simulink subsystem "ClusteringAlgoTemplate"  (R2022b)
settings: Solver=VariableStepAuto  StartTime=0.0  StopTime=10.0  RelTol=1e-3
settings Model: Creator=smryk  LastModifiedBy=smryk

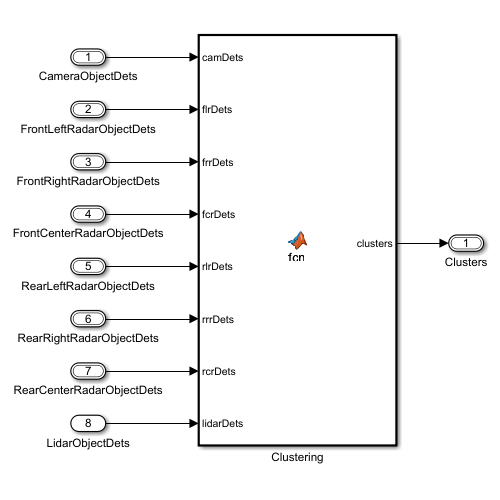
[thumbnail: Simulink's stored preview of the top-level diagram]
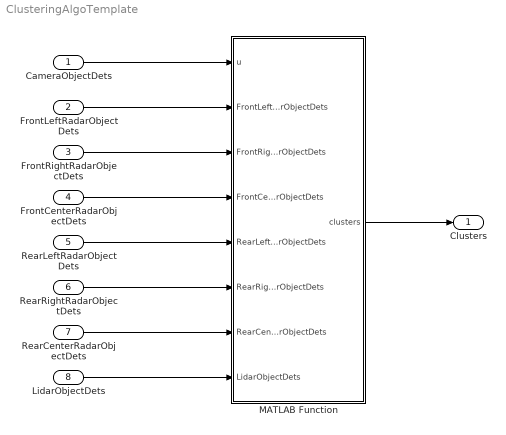
== system ClusteringAlgoTemplate ==
  CameraObjectDets : Inport  OutDataTypeStr=Bus: BusObjectDetections1
  FrontLeftRadarObjectDets : Inport  Port=2  OutDataTypeStr=Bus: BusDrivingRadarDataGenerator1
  FrontRightRadarObjectDets : Inport  Port=3  OutDataTypeStr=Bus: BusDrivingRadarDataGenerator1
  FrontCenterRadarObjectDets : Inport  Port=4  OutDataTypeStr=Bus: BusDrivingRadarDataGenerator1
  RearLeftRadarObjectDets : Inport  Port=5  OutDataTypeStr=Bus: BusDrivingRadarDataGenerator1
  RearRightRadarObjectDets : Inport  Port=6  OutDataTypeStr=Bus: BusDrivingRadarDataGenerator1
  RearCenterRadarObjectDets : Inport  Port=7  OutDataTypeStr=Bus: BusDrivingRadarDataGenerator1
  LidarObjectDets : Inport  Port=8
  MATLAB Function : MATLAB Function  TreatAsAtomicUnit=on
  Clusters : Outport  OutDataTypeStr=Bus: BusObjectDetections1
  wires:
  LidarObjectDets/1 -> MATLAB Function/8(LidarObjectDets)
  RearCenterRadarObjectDets/1 -> MATLAB Function/7(RearCenterRadarObjectDets)
  RearRightRadarObjectDets/1 -> MATLAB Function/6(RearRightRadarObjectDets)
  RearLeftRadarObjectDets/1 -> MATLAB Function/5(RearLeftRadarObjectDets)
  FrontCenterRadarObjectDets/1 -> MATLAB Function/4(FrontCenterRadarObjectDets)
  FrontRightRadarObjectDets/1 -> MATLAB Function/3(FrontRightRadarObjectDets)
  FrontLeftRadarObjectDets/1 -> MATLAB Function/2(FrontLeftRadarObjectDets)
  MATLAB Function/1(clusters) -> Clusters/1
  CameraObjectDets/1 -> MATLAB Function/1(u)

== matlab function ClusteringAlgoTemplate/MATLAB Function ==
  data: u input; clusters output Bus: BusObjectDetections1; FrontLeftRadarObjectDets input; FrontRightRadarObjectDets input; FrontCenterRadarObjectDets input; RearLeftRadarObjectDets input; RearRightRadarObjectDets input; RearCenterRadarObjectDets input; LidarObjectDets input
function clusters = fcn(u, FrontLeftRadarObjectDets, FrontRightRadarObjectDets, FrontCenterRadarObjectDets, RearLeftRadarObjectDets, RearRightRadarObjectDets, RearCenterRadarObjectDets, LidarObjectDets)

clusters.NumDetections = 0;
clusters.IsValidTime = boolean(0);

fakeMeasurementParams.Frame = drivingCoordinateFrameType(0);
fakeMeasurementParams.OriginPosition = [0; 0; 0];
fakeMeasurementParams.Orientation = [0 0 0; 0 0 0; 0 0 0];
fakeMeasurementParams.HasVelocity = boolean(0);

fakeObjAttributes.TargetIndex = 0;

fakeDetection.Time = 0;
fakeDetection.Measurement = [0; 0; 0; 0; 0; 0];
fakeDetection.MeasurementNoise = [0 0 0 0 0 0; 0 0 0 0 0 0; 0 0 0 0 0 0; 0 0 0 0 0 0; 0 0 0 0 0 0; 0 0 0 0 0 0];
fakeDetection.SensorIndex = 0;
fakeDetection.ObjectClassID = 0;
fakeDetection.MeasurementParameters = fakeMeasurementParams;
fakeDetection.ObjectAttributes = fakeObjAttributes;

for i = 1:50
    clusters.Detections(i) = fakeDetection;
end
